simulink model "StSys_StrtBas"  (R2016b)
settings: configuration reference "CodeGenConfigSet" (kept outside this file)
values from neighbouring files (symbols this model uses):
  StSys_nAdjMax_C = Calibration.Parameter    [init_StSys_StrtBas.m]    (also in init_StSys_StrtBas_SIL.m = Simulink.Parameter)
  StSys_trqAdjMax_C = Calibration.Parameter    [init_StSys_StrtBas.m]    (also in init_StSys_StrtBas_SIL.m = Simulink.Parameter)
  StSys_trqStrtBas_MAP = Calibration.Parameter    [init_StSys_StrtBas.m]    (also in init_StSys_StrtBas_SIL.m = Simulink.Parameter)
  StSys_trqStrtBas_MAPX = Calibration.Parameter    [init_StSys_StrtBas.m]    (also in init_StSys_StrtBas_SIL.m = Simulink.Parameter)
  StSys_trqStrtBas_MAPY = Calibration.Parameter    [init_StSys_StrtBas.m]    (also in init_StSys_StrtBas_SIL.m = Simulink.Parameter)
  TRQ_ZERO = fi(0,Trq_Nm)    [init_StSys_StrtBas.m]    (also in init_StSys_StrtBas_SIL.m)
libraries: CXLib x1
settings Model: Creator=Colin  LastModifiedBy=lenovo
settings ConfigSetRef: SourceLocation=Base Workspace

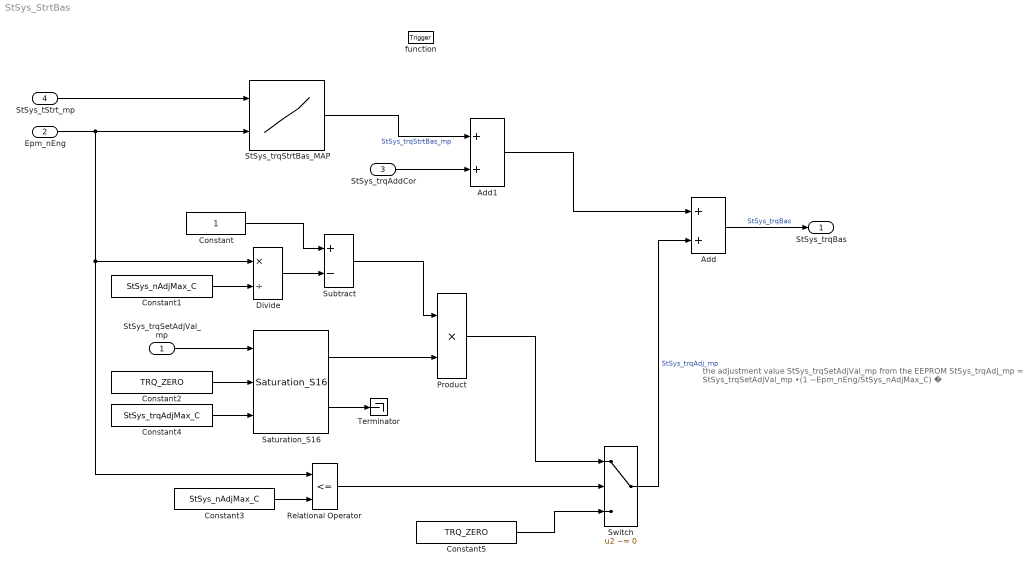
== system StSys_StrtBas ==
  note: the adjustment value StSys_trqSetAdjVal_mp from the EEPROM
      |
      | StSys_trqAdj_mp = StSys_trqSetAdjVal_mp •(1 −Epm_nEng/StSys_nAdjMax_C)
      | �
  StSys_trqSetAdjVal_mp : Inport  Tag=Nm  Description=EPPROM adjustment value for start torque correction  OutMin=0  OutMax=1000  OutDataTypeStr=Trq_Nm
  Epm_nEng : Inport  Tag=rpm  Description=Engine speed  Port=2  OutMin=0  OutMax=6000  OutDataTypeStr=EngSpeed_rpm
  StSys_trqAddCor : Inport  Tag=Nm  Description=additional correction torque for starting torque  Port=3  OutMin=0  OutMax=1000  OutDataTypeStr=Trq_Nm
  StSys_tStrt_mp : Inport  Tag=deg  Description=engine temperature for starting system  Port=4  OutMin=-50  OutMax=150  OutDataTypeStr=Temp_deg
  function : TriggerPort  TriggerType=function-call  VariantControl=Variant
  Add : Sum  SaturateOnIntegerOverflow=on
  Add1 : Sum
  Constant : Constant  OutDataTypeStr=Inherit: Inherit via back propagation
  Constant1 : Constant  Value=StSys_nAdjMax_C
  Constant2 : Constant  Value=TRQ_ZERO  OutDataTypeStr=Trq_Nm
  Constant3 : Constant  Value=StSys_nAdjMax_C
  Constant4 : Constant  Value=StSys_trqAdjMax_C
  Constant5 : Constant  Value=TRQ_ZERO  OutDataTypeStr=Trq_Nm
  Divide : Product  Inputs=*/  OutDataTypeStr=Factor
  Product : Product  OutDataTypeStr=Trq_Nm  SaturateOnIntegerOverflow=on
  Relational Operator : RelationalOperator  Operator=<=  OutDataTypeStr=boolean  RndMeth=Simplest
  Saturation_S16 : CXLib/Saturation_S16
  StSys_trqStrtBas_MAP : Lookup_n-D  BreakpointsForDimension1=StSys_trqStrtBas_MAPY  BreakpointsForDimension2=StSys_trqStrtBas_MAPX  IndexSearchMethod=Linear search  BeginIndexSearchUsingPreviousIndexResult=on  Table=StSys_trqStrtBas_MAP  ExtrapMethod=Clip  UseLastTableValue=on  InternalRulePriority=Speed  OutDataTypeStr=Inherit: Inherit from 'Table data'  RndMeth=Simplest  SaturateOnIntegerOverflow=on
  Subtract : Sum  Inputs=+-  OutDataTypeStr=Inherit: Inherit via back propagation
  Switch : Switch  Criteria=u2 ~= 0  InputSameDT=on
  Terminator : Terminator
  StSys_trqBas : Outport  Tag=Nm  Description=basic starting torque  OutMin=0  OutMax=1000  OutDataTypeStr=Trq_Nm
  wires:
  Epm_nEng/1 -> StSys_trqStrtBas_MAP/2, Relational Operator/1, Divide/1
  StSys_trqStrtBas_MAP/1 -> Add1/1  "StSys_trqStrtBas_mp"
  StSys_trqAddCor/1 -> Add1/2
  Add/1 -> StSys_trqBas/1  "StSys_trqBas"
  Add1/1 -> Add/1
  StSys_trqSetAdjVal_mp/1 -> Saturation_S16/1
  Saturation_S16/2 -> Terminator/1
  Divide/1 -> Subtract/2
  Constant/1 -> Subtract/1
  Constant1/1 -> Divide/2
  Constant2/1 -> Saturation_S16/2
  Constant4/1 -> Saturation_S16/3
  Constant3/1 -> Relational Operator/2
  Relational Operator/1 -> Switch/2
  Constant5/1 -> Switch/3
  Switch/1 -> Add/2  "StSys_trqAdj_mp"
  Subtract/1 -> Product/1
  Saturation_S16/1 -> Product/2
  Product/1 -> Switch/1
  StSys_tStrt_mp/1 -> StSys_trqStrtBas_MAP/1
